simulink model "SG_direct_DLE_position_control_hose_pump_v2"  (R2025b)
settings: Solver=FixedStepAuto  StartTime=0.0  StopTime=inf  FixedStep=0.0001  RelTol=1e-3
undefined symbols (not defined in the file): DiscIntNeverNeededParam
libraries: slrealtimeloglib x8, simulink x4, slrealtimeseriallib x3, SG_DLE_position_control_module_hose_pump x1, servo_valve_pressure_control_module x1
settings Model: Creator=cmmcguir  LastModifiedBy=cmmcguir
settings SolverCC: ConcurrentTasks=on  PositivePriorityOrder=on
settings OptimizationCC: BlockReduction=off  OptimizeBlockIOStorage=off
settings DebuggingCC: TasksWithSamePriorityMsg=none
settings HardwareCC: ProdBitPerLong=64.0  ProdLongLongMode=on  ProdHWDeviceType=Intel->x86-64 (Linux 64)
settings RTWCC: SystemTargetFile=speedgoat.tlc  TemplateMakefile=slrealtime_default_tmf  Toolchain=Simulink Real-Time Toolchain  BuildConfiguration=Faster Runs  CodeExecutionProfiling=on  TargetLang=C++  Description=Speedgoat Real-Time Target Machine
settings SimulinkRealTimeTargetCC: SLRTFileLogMaxRuns=3.0  ExtModeMaxTrigDuration=10.0  ExtModeStaticAllocSize=1000000.0  ExtModeTransport=0.0  MultiwordLength=2048.0  DynamicStringBufferSize=256.0  PreserveMATLABNamespacesInGeneratedCode=on  SubcomponentCodeInterfacePackaging=Reusable function  MATLABClassNameForMDSCustomization=Simulink.SoftwareTarget.GRTCustomization  InstructionSetFMA=off  LogToMDFFile=off

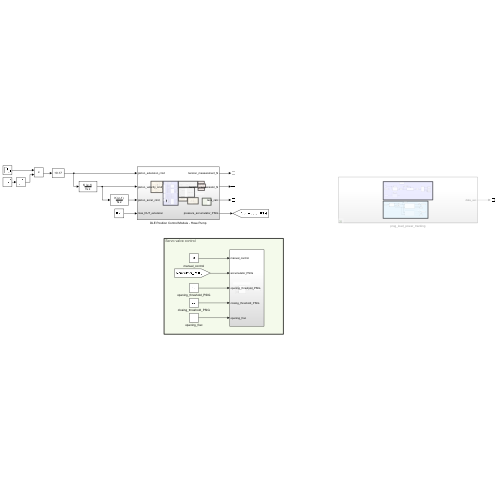
[thumbnail: Simulink's stored preview of the top-level diagram]
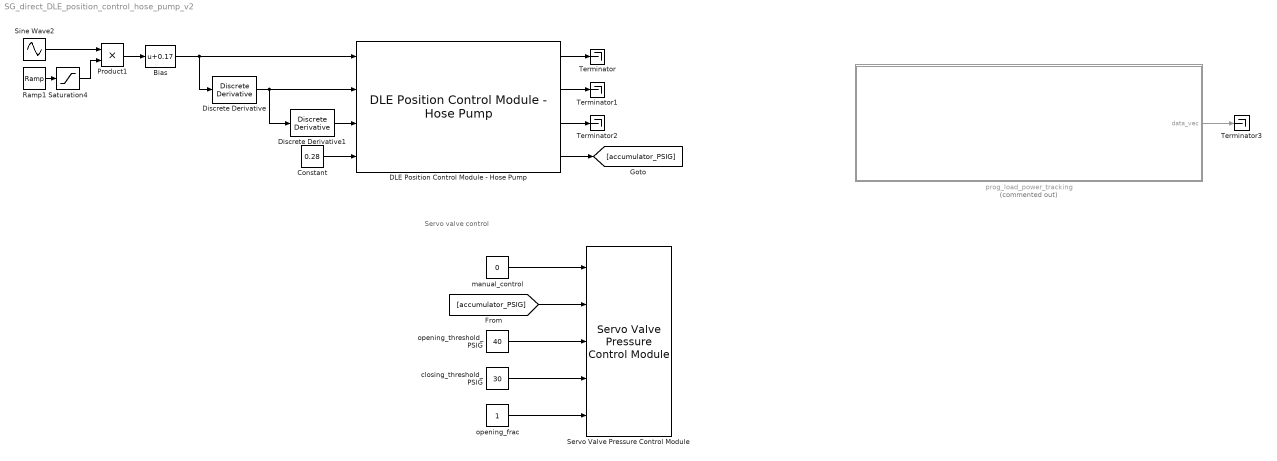
== system SG_direct_DLE_position_control_hose_pump_v2 ==
  note: Servo valve control
  Bias : Bias  Bias=0.17  SaturateOnIntegerOverflow=off
  Constant : Constant  Value=0.28
  DLE Position Control Module - Hose Pump : SG_DLE_position_control_module_hose_pump/DLE Position Control Module - Hose Pump  SystemSampleTime=-1  VariantActivationTime=update diagram  EmptyChoice=off  PassThrough=off  PassThroughVariantControl=(default)  EmptyChoiceVariantControl=(default)  AllowFlexibleInterface=on  Latency=0  AutoFrameSizeCalculation=off
  Discrete Derivative : simulink/Discrete/Discrete Derivative  gainval=1.0  ICPrevScaledInput=0.0  OutMin=[]  OutMax=[]  OutDataType=fixdt(1, 16)  OutScaling=2^-10  DoSatur=off
  Discrete Derivative1 : simulink/Discrete/Discrete Derivative  gainval=1.0  ICPrevScaledInput=0.0  OutMin=[]  OutMax=[]  OutDataType=fixdt(1, 16)  OutScaling=2^-10  DoSatur=off
  Product1 : Product
  Ramp1 : simulink/Sources/Ramp  slope=1/10  start=10  InitialOutput=0
  Saturation4 : Saturate  UpperLimit=1  LowerLimit=0
  Servo Valve Pressure Control Module : servo_valve_pressure_control_module/Servo Valve Pressure Control Module  SystemSampleTime=-1  VariantActivationTime=update diagram  EmptyChoice=off  PassThrough=off  PassThroughVariantControl=(default)  EmptyChoiceVariantControl=(default)  AllowFlexibleInterface=on  Latency=0  AutoFrameSizeCalculation=off
  Sine Wave2 : Sin  Amplitude=0.05  Frequency=2*pi/5  SampleTime=0.0001
  Terminator{,1..3} (4 alike) : Terminator
  closing_threshold_PSIG : Constant  Value=30
  manual_control : Constant  Value=0  SampleTime=0.0001
  opening_frac : Constant
  opening_threshold_PSIG : Constant  Value=40
  prog_load_power_tracking : Subsystem  Commented=on
  wires:
  Constant/1 -> DLE Position Control Module - Hose Pump/4
  Sine Wave2/1 -> Product1/1
  Product1/1 -> Bias/1
  Saturation4/1 -> Product1/2
  Discrete Derivative1/1 -> DLE Position Control Module - Hose Pump/3
  Ramp1/1 -> Saturation4/1
  Bias/1 -> DLE Position Control Module - Hose Pump/1, Discrete Derivative/1
  Discrete Derivative/1 -> DLE Position Control Module - Hose Pump/2, Discrete Derivative1/1
  opening_frac/1 -> Servo Valve Pressure Control Module/5
  opening_threshold_PSIG/1 -> Servo Valve Pressure Control Module/3
  manual_control/1 -> Servo Valve Pressure Control Module/1
  closing_threshold_PSIG/1 -> Servo Valve Pressure Control Module/4
  [accumulator_PSIG] -> Servo Valve Pressure Control Module/2
  DLE Position Control Module - Hose Pump/1 -> Terminator/1
  DLE Position Control Module - Hose Pump/2 -> Terminator1/1
  DLE Position Control Module - Hose Pump/3 -> Terminator2/1
  DLE Position Control Module - Hose Pump/4 -> [accumulator_PSIG]
  prog_load_power_tracking/1(data_vec) -> Terminator3/1

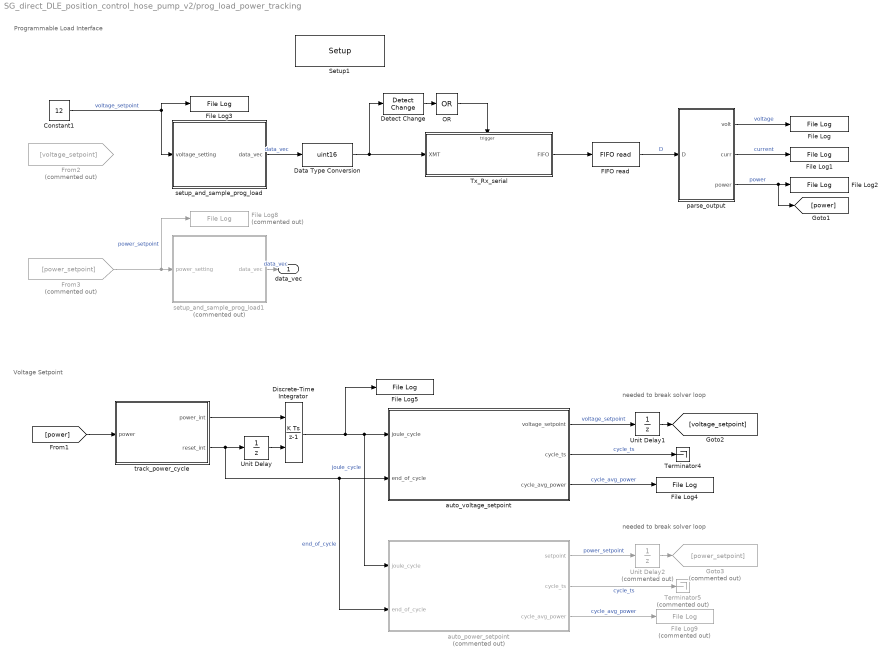
== system SG_direct_DLE_position_control_hose_pump_v2/prog_load_power_tracking ==
  note: needed to break solver loop
  note: Programmable Load Interface
  note: needed to break solver loop
  note: Voltage Setpoint
  Constant1 : Constant  Value=12
  Data Type Conversion : DataTypeConversion  OutDataTypeStr=uint16  SaturateOnIntegerOverflow=off  RndMeth=Floor
  Detect Change : simulink/Logic and Bit Operations/Detect Change  vinit=0  OutDataTypeStr=boolean
  Discrete-Time Integrator : DiscreteIntegrator  ExternalReset=rising  SampleTime=-1  ICPrevOutput=DiscIntNeverNeededParam  ICPrevScaledInput=DiscIntNeverNeededParam
  FIFO read : slrealtimeseriallib/FIFO read  maxsize=16  minsize=1  usedelimiter=on  delimiter=10  outputtype=8 bit uint null terminated  enable=off  enableout=off  sampletime=-1
  File Log{,1..5} (6 alike) : slrealtimeloglib/File Log  decimation=1  inputProcessing=Elements as channels (sample based)
  File Log8 : slrealtimeloglib/File Log  Commented=on  decimation=1  inputProcessing=Elements as channels (sample based)
  File Log9 : slrealtimeloglib/File Log  Commented=on  decimation=1  inputProcessing=Elements as channels (sample based)
  From2 : From  Commented=on  GotoTag=voltage_setpoint
  From3 : From  Commented=on  GotoTag=power_setpoint
  Goto3 : Goto  Commented=on  GotoTag=power_setpoint
  OR : Logic  Operator=OR  Inputs=1  IconShape=distinctive  AllPortsSameDT=off  OutDataTypeStr=boolean
  Setup1 : slrealtimeseriallib/Mainboard/Setup  port=USB Serial Port 2  baud=115200  width=8  nstop=1  parity=None  ctsmode=on
  Terminator4 : Terminator
  Terminator5 : Terminator  Commented=on
  Tx_Rx_serial : Subsystem
  Unit Delay : UnitDelay  SampleTime=-1  HasFrameUpgradeWarning=on
  Unit Delay1 : UnitDelay  SampleTime=-1  HasFrameUpgradeWarning=on
  Unit Delay2 : UnitDelay  Commented=on  SampleTime=-1  HasFrameUpgradeWarning=on
  auto_power_setpoint : Stateflow chart  Commented=on  TreatAsAtomicUnit=on  SystemSampleTime=0.001
  auto_voltage_setpoint : Stateflow chart  TreatAsAtomicUnit=on  SystemSampleTime=0.001
  parse_output : MATLAB Function  TreatAsAtomicUnit=on
  setup_and_sample_prog_load : Test Sequence  TreatAsAtomicUnit=on  SystemSampleTime=0.001
  setup_and_sample_prog_load1 : Test Sequence  Commented=on  TreatAsAtomicUnit=on  SystemSampleTime=0.001
  track_power_cycle : Stateflow chart  TreatAsAtomicUnit=on
  data_vec : Outport
  wires:
  auto_voltage_setpoint/3(cycle_avg_power) -> File Log4/1  "cycle_avg_power"
  Constant1/1 -> setup_and_sample_prog_load/1(voltage_setting), File Log3/1  "voltage_setpoint"
  Tx_Rx_serial/1(FIFO) -> FIFO read/1
  Detect Change/1 -> OR/1
  OR/1 -> Tx_Rx_serial/Trigger
  Unit Delay1/1 -> [voltage_setpoint]
  parse_output/1(volt) -> File Log/1  "voltage"
  [power] -> track_power_cycle/1(power)
  FIFO read/1 -> parse_output/1(D)  "D"
  parse_output/3(power) -> [power], File Log2/1  "power"
  auto_power_setpoint/2(cycle_ts) -> Terminator5/1  "cycle_ts"
  From3/1 -> setup_and_sample_prog_load1/1(power_setting), File Log8/1  "power_setpoint"
  track_power_cycle/2(reset_int) -> auto_power_setpoint/2(end_of_cycle), auto_voltage_setpoint/2(end_of_cycle), Unit Delay/1  "end_of_cycle"
  track_power_cycle/1(power_int) -> Discrete-Time Integrator/1
  auto_power_setpoint/3(cycle_avg_power) -> File Log9/1  "cycle_avg_power"
  setup_and_sample_prog_load/1(data_vec) -> Data Type Conversion/1  "data_vec"
  Data Type Conversion/1 -> Detect Change/1, Tx_Rx_serial/1(XMT)
  Discrete-Time Integrator/1 -> File Log5/1, auto_power_setpoint/1(joule_cycle), auto_voltage_setpoint/1(joule_cycle)  "joule_cycle"
  setup_and_sample_prog_load1/1(data_vec) -> data_vec/1  "data_vec"
  auto_voltage_setpoint/2(cycle_ts) -> Terminator4/1  "cycle_ts"
  auto_power_setpoint/1(setpoint) -> Unit Delay2/1  "power_setpoint"
  Unit Delay/1 -> Discrete-Time Integrator/2
  auto_voltage_setpoint/1(voltage_setpoint) -> Unit Delay1/1  "voltage_setpoint"
  parse_output/2(curr) -> File Log1/1  "current"
  Unit Delay2/1 -> Goto3/1

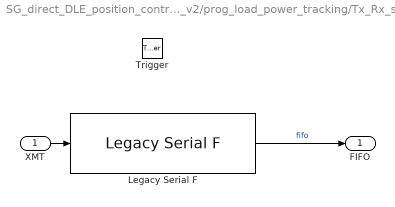
== system SG_direct_DLE_position_control_hose_pump_v2/prog_load_power_tracking/Tx_Rx_serial ==
  XMT : Inport
  Trigger : TriggerPort  VariantControl=(inherit)  PortDimensions=1
  Legacy Serial F : slrealtimeseriallib/Mainboard/Legacy Serial F  port=USB Serial Port 2  baud=115200  width=8  nstop=1  parity=None  ctsmode=off  fifosize=16  idtype=count+16 bit uint  sampletime=-1
  FIFO : Outport
  wires:
  XMT/1 -> Legacy Serial F/1
  Legacy Serial F/1 -> FIFO/1  "fifo"

== stateflow chart SG_direct_DLE_position_control_hose_pump_v2/prog_load_power_tracking/track_power_cycle ==
  state zero_pow
    en, du:
    power_int = 0;
    du:
    reset_int = false;
  state timeout
    en, du:
    power_int = power;
  state pos_pow
    en, du:
    power_int = power;
  (default) -> zero_pow
  zero_pow -> pos_pow : [power >= 0.005]
  timeout -> zero_pow [order 2] : [after(0.5, sec)] % need at least
      |  % two samples of power less than 5 mW
      | {reset_int = true;}
  timeout -> pos_pow [order 1] : [power >= 0.005]
  pos_pow -> timeout : [power < 0.005]
  data: power input; power_int output; reset_int output boolean size=1

== stateflow chart SG_direct_DLE_position_control_hose_pump_v2/prog_load_power_tracking/setup_and_sample_prog_load ==
  state step_1 % hold
    data_vec = zeros(64, 1);
  state step_2 % set operating condition - CV
    data_vec(1) = 17; % length of message + CR LF
    data_vec(2:7) = [58 86 79 76 84 32];
    volt_set = zeros(1, 8);
    sprf_len = length(sprintf('%.3f', voltage_setting));
    volt_set(1:sprf_len) = double(sprintf('%.3f', voltage_setting));
    if sprf_len < 8
    volt_set(sprf_len+1 : 8) = 48;
    end
    data_vec(8:15) = volt_set;
    data_vec(16:18) = [86 13 10]; % 'V' CR LF
  state step_3 % enable device
    data_vec(1) = 9; % length of message + CR LF
    data_vec(2:8) = [58 73 78 80 32 79 78];
    data_vec(9:10) = [13 10]; % CRLF
  state step_4 % take voltage reading
    data_vec(1) = 13; % length of message + CR LF
    data_vec(2:12) = [58 77 69 65 83 58 86 79 76 84 63];
    data_vec(13:14) = [13 10]; % CRLF
  state step_5 % take current reading
    data_vec(1) = 13; % length of message + CR LF
    data_vec(2:12) = [58 77 69 65 83 58 67 85 82 82 63];
    data_vec(13:14) = [13 10]; % CRLF
  state step_6 % take power reading
    data_vec(1) = 12; % length of message + CR LF
    data_vec(2:11) = [58 77 69 65 83 58 80 79 87 63];
    data_vec(12:13) = [13 10]; % CRLF
  state step_7 % set operating condition - CV
    data_vec(1) = 17; % length of message + CR LF
    data_vec(2:7) = [58 86 79 76 84 32];
    volt_set = zeros(1, 8);
    sprf_len = length(sprintf('%.3f', voltage_setting));
    volt_set(1:sprf_len) = double(sprintf('%.3f', voltage_setting));
    if sprf_len < 8
    volt_set(sprf_len+1 : 8) = 48;
    end
    data_vec(8:15) = volt_set;
    data_vec(16:18) = [86 13 10]; % 'V' CR LF
  (default) -> step_1 % hold
  step_1 % hold -> step_2 % set operating condition - CV : [
      | after(1, sec)
      | ]
  step_2 % set operating condition - CV -> step_3 % enable device : [
      | after(1, sec)
      | ]
  step_3 % enable device -> step_4 % take voltage reading : [
      | after(1, sec)
      | ]
  (junction 46) -> step_4 % take voltage reading
  (junction 48) -> (junction 46)
  step_4 % take voltage reading -> step_5 % take current reading : [
      | after(0.01, sec)
      | ]
  step_5 % take current reading -> step_6 % take power reading : [
      | after(0.01, sec)
      | ]
  step_6 % take power reading -> step_7 % set operating condition - CV : [
      | after(0.01, sec)
      | ]
  step_7 % set operating condition - CV -> (junction 48) : [
      | after(0.07, sec)
      | ]
  data: data_vec output size=[64 1] =zeros(64, 1); voltage_setting input; volt_set local size=[1 8]; sprf_len local

== stateflow chart SG_direct_DLE_position_control_hose_pump_v2/prog_load_power_tracking/setup_and_sample_prog_load1 ==
  state step_1 % hold
    data_vec = zeros(64, 1);
  state step_2 % set operating condition - CW
    data_vec(1) = 16; % length of message + CR LF
    data_vec(2:6) = [58    80    79    87    32];
    power_set = zeros(1, 8);
    sprf_len = length(sprintf('%.3f', power_setting));
    power_set(1:sprf_len) = double(sprintf('%.3f', power_setting));
    if sprf_len < 8
    power_set(sprf_len+1 : 8) = 48;
    end
    data_vec(7:14) = power_set;
    data_vec(15:17) = [87 13 10]; % 'W' CR LF
  state step_3 % enable device
    data_vec(1) = 9; % length of message + CR LF
    data_vec(2:8) = [58 73 78 80 32 79 78];
    data_vec(9:10) = [13 10]; % CRLF
  state step_4 % take voltage reading
    data_vec(1) = 13; % length of message + CR LF
    data_vec(2:12) = [58 77 69 65 83 58 86 79 76 84 63];
    data_vec(13:14) = [13 10]; % CRLF
  state step_5 % take current reading
    data_vec(1) = 13; % length of message + CR LF
    data_vec(2:12) = [58 77 69 65 83 58 67 85 82 82 63];
    data_vec(13:14) = [13 10]; % CRLF
  state step_6 % take power reading
    data_vec(1) = 12; % length of message + CR LF
    data_vec(2:11) = [58 77 69 65 83 58 80 79 87 63];
    data_vec(12:13) = [13 10]; % CRLF
  state step_7 % set operating condition - CW
    data_vec(1) = 16; % length of message + CR LF
    data_vec(2:6) = [58    80    79    87    32];
    power_set = zeros(1, 8);
    sprf_len = length(sprintf('%.3f', power_setting));
    power_set(1:sprf_len) = double(sprintf('%.3f', power_setting));
    if sprf_len < 8
    power_set(sprf_len+1 : 8) = 48;
    end
    data_vec(7:14) = power_set;
    data_vec(15:17) = [87 13 10]; % 'W' CR LF
  (default) -> step_1 % hold
  step_1 % hold -> step_2 % set operating condition - CW : [
      | after(1, sec)
      | ]
  step_2 % set operating condition - CW -> step_3 % enable device : [
      | after(1, sec)
      | ]
  step_3 % enable device -> step_4 % take voltage reading : [
      | after(1, sec)
      | ]
  (junction 46) -> step_4 % take voltage reading
  (junction 48) -> (junction 46)
  step_4 % take voltage reading -> step_5 % take current reading : [
      | after(0.01, sec)
      | ]
  step_5 % take current reading -> step_6 % take power reading : [
      | after(0.01, sec)
      | ]
  step_6 % take power reading -> step_7 % set operating condition - CW : [
      | after(0.01, sec)
      | ]
  step_7 % set operating condition - CW -> (junction 48) : [
      | after(0.07, sec)
      | ]
  data: data_vec output size=[64 1] =zeros(64, 1); power_setting input; power_set local size=[1 8]; sprf_len local

== stateflow chart SG_direct_DLE_position_control_hose_pump_v2/prog_load_power_tracking/auto_power_setpoint ==
  state init
    en:
    setpoint = starting_set;
    setpoint_best = setpoint;
    perf_buffer = zeros(1, num_cycles_per_update);
  state monitor_cycle
    en:
    cycle_ts(1) = cycle_ts(2); % [cycle_start_ts, end_ts]
  state calc_cycle_avg_power
    en:
    cycle_ts(2) = t; % [cycle_start_ts, end_ts]
    % cycle_avg_power = joule_cycle / (cycle_ts(2) - cycle_ts(1));
    perf_buffer(perf_buffer_ind) = joule_cycle / (cycle_ts(2) - cycle_ts(1));
    perf_buffer_ind = perf_buffer_ind + 1;
  state check_for_improvement
    en:
    avg_power_buffer(2) = avg_power_buffer(1);
    cycle_avg_power = mean(perf_buffer);
    avg_power_buffer(1) = cycle_avg_power;
    perf_buffer_ind = 1;
    perf_buffer = zeros(1, num_cycles_per_update);
    %
    %  check if power was improved
    if avg_power_buffer(1) > avg_power_buffer(2) % improvement
    setpoint_best = setpoint; % record best
    setpoint = setpoint + setpoint_delta; % disturb
    else % worsened or the same
    setpoint_delta = 0.5 * setpoint_delta;
    setpoint = setpoint_best + setpoint_delta; % disturb by half dV
    end
    setpoint = min([max([setpoint, min_set]), max_set]);
  (default) -> init
  init -> monitor_cycle : [end_of_cycle] {cycle_ts(2) = t;}
  (junction 36) -> monitor_cycle
  (junction 35) -> (junction 36)
  monitor_cycle -> calc_cycle_avg_power : [end_of_cycle]
  calc_cycle_avg_power -> (junction 35) [order 2]
  (junction 45) -> (junction 35)
  calc_cycle_avg_power -> check_for_improvement [order 1] : [perf_buffer_ind > num_cycles_per_update]
  check_for_improvement -> (junction 45)
  data: joule_cycle input; end_of_cycle input; starting_set constant double size=1 =0.01; setpoint output; min_set constant double =0.01; max_set constant double =10; cycle_ts output size=[1 2] =[0 0]; cycle_avg_power output size=1; avg_power_buffer local size=[1 2] =zeros(1, 2); setpoint_best local; setpoint_delta local =0.01; perf_buffer local; perf_buffer_ind local size=1 =1; num_cycles_per_update constant double size=1 =3

== stateflow chart SG_direct_DLE_position_control_hose_pump_v2/prog_load_power_tracking/auto_voltage_setpoint ==
  state init
    en:
    voltage_setpoint = starting_volt_set;
    voltage_setpoint_best = voltage_setpoint;
    perf_buffer = zeros(1, num_cycles_per_update);
  state monitor_cycle
    en:
    cycle_ts(1) = cycle_ts(2); % [cycle_start_ts, end_ts]
  state calc_cycle_avg_power
    en:
    cycle_ts(2) = t; % [cycle_start_ts, end_ts]
    % cycle_avg_power = joule_cycle / (cycle_ts(2) - cycle_ts(1));
    perf_buffer(perf_buffer_ind) = joule_cycle / (cycle_ts(2) - cycle_ts(1));
    perf_buffer_ind = perf_buffer_ind + 1;
  state check_for_improvement
    en:
    avg_power_buffer(2) = avg_power_buffer(1);
    cycle_avg_power = mean(perf_buffer);
    avg_power_buffer(1) = cycle_avg_power;
    perf_buffer_ind = 1;
    perf_buffer = zeros(1, num_cycles_per_update);
    %
    %  check if power was improved
    if avg_power_buffer(1) > avg_power_buffer(2) % improvement
    voltage_setpoint_best = voltage_setpoint; % record best
    voltage_setpoint = voltage_setpoint + voltage_setpoint_dV; % disturb
    else % worsened or the same
    %voltage_setpoint_dV = 0.5 * voltage_setpoint_dV;
    %voltage_setpoint = voltage_setpoint_best - voltage_setpoint_dV; % step back
    voltage_setpoint_dV = -0.5 * voltage_setpoint_dV;
    voltage_setpoint = voltage_setpoint + voltage_setpoint_dV; % step back
    end
    voltage_setpoint = min([max([voltage_setpoint, min_voltage_set]), max_voltage_set]);
  (default) -> init
  init -> monitor_cycle : [end_of_cycle] {cycle_ts(2) = t;}
  (junction 36) -> monitor_cycle
  (junction 35) -> (junction 36)
  monitor_cycle -> calc_cycle_avg_power : [end_of_cycle]
  calc_cycle_avg_power -> (junction 35) [order 2]
  (junction 45) -> (junction 35)
  calc_cycle_avg_power -> check_for_improvement [order 1] : [perf_buffer_ind > num_cycles_per_update]
  check_for_improvement -> (junction 45)
  data: joule_cycle input; end_of_cycle input; starting_volt_set constant double size=1 =2; voltage_setpoint output; min_voltage_set constant double =1; max_voltage_set constant double =10; cycle_ts output size=[1 2] =[0 0]; cycle_avg_power output size=1; avg_power_buffer local size=[1 2] =zeros(1, 2); voltage_setpoint_best local; voltage_setpoint_dV local =1; perf_buffer local; perf_buffer_ind local size=1 =1; num_cycles_per_update constant double size=1 =5

== matlab function SG_direct_DLE_position_control_hose_pump_v2/prog_load_power_tracking/parse_output ==
  data: D input; volt output; curr output; power output
function [volt, curr, power] = fcn(D)

persistent volt_pers
persistent curr_pers
persistent power_pers

if isempty(volt_pers) % set persistent variable values
    volt_pers = 0;
    curr_pers = 0;
    power_pers = 0;
end

if D(1) ~= 0
    switch D(7)
        case 86 % 'V' --> voltage reading
            volt_pers = real(str2double(char(D(1:6))));
        case 87 % 'W' --> power reading
            power_pers = real(str2double(char(D(1:6))));
        case 65 % 'A' --> current reading
            curr_pers = real(str2double(char(D(1:6))));
    end
end

% output
volt = volt_pers;
curr = curr_pers;
power = power_pers;
